simulink model "time_variant_invariant_system_ex1"  (R2018b)
settings: Solver=FixedStepAuto  StartTime=0.0  StopTime=10  FixedStep=1e-3  RelTol=1e-3
settings Model: Creator=auralius  LastModifiedBy=auralius

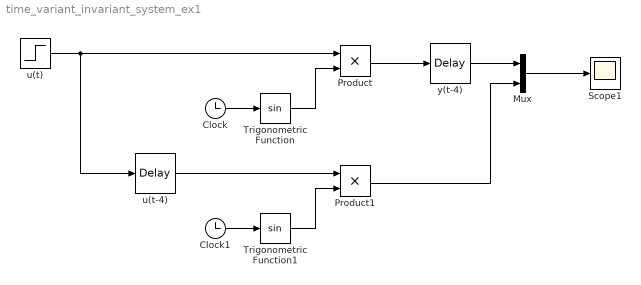
== system time_variant_invariant_system_ex1 ==
  Clock : Clock
  Clock1 : Clock
  Mux : Mux  Inputs=2
  Product : Product
  Product1 : Product
  Scope1 : Scope
  Trigonometric Function : Trigonometry
  Trigonometric Function1 : Trigonometry
  u(t) : Step
  u(t-4) : TransportDelay  DelayTime=4
  y(t-4) : TransportDelay  DelayTime=4
  wires:
  u(t-4)/1 -> Product1/1
  u(t)/1 -> u(t-4)/1, Product/1
  y(t-4)/1 -> Mux/1
  Mux/1 -> Scope1/1
  Clock/1 -> Trigonometric Function/1
  Trigonometric Function/1 -> Product/2
  Trigonometric Function1/1 -> Product1/2
  Clock1/1 -> Trigonometric Function1/1
  Product/1 -> y(t-4)/1
  Product1/1 -> Mux/2
